simulink model "switch_detect"  (R2023a)
settings: configuration reference "config" (kept outside this file)
model workspace (MAT data in the model file):
  switch_pos = Simulink.Parameter
  switch_pos.Value = 10000
  switch_pos.Description = '开关触发时刻编码器位置'
  switch_pos.DataType = 'int32'
  switch_pos.Complexity = 'real'
  switch_pos.Dimensions = [1 1]
  switch_width = Simulink.Parameter
  switch_width.Value = 10
  switch_width.Description = '开关触发宽度
    | '
  switch_width.DataType = 'int32'
  switch_width.Min = 0
  switch_width.Complexity = 'real'
  switch_width.Dimensions = [1 1]
libraries: servo_hub_lib x1
settings Model: DataDictionary=model_config.sldd  ParameterArgumentNames=switch_pos,switch_width  Creator=huangcheng  LastModifiedBy=Administrator
settings ConfigSetRef: SourceName=config

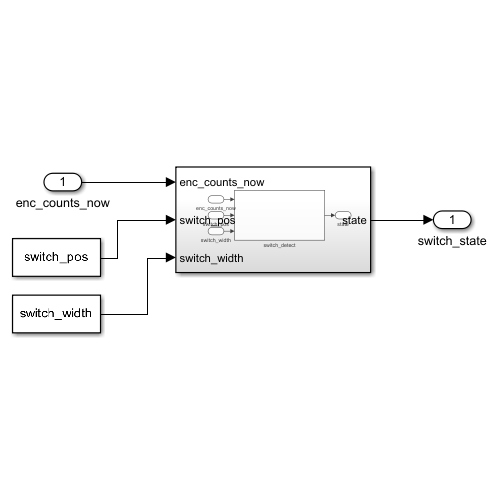
[thumbnail: Simulink's stored preview of the top-level diagram]
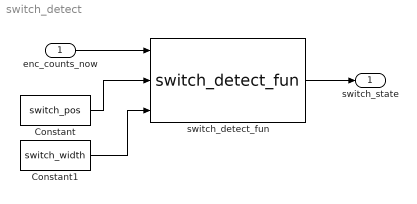
== system switch_detect ==
  enc_counts_now : Inport  OutDataTypeStr=int64
  Constant : Constant  Value=switch_pos  SampleTime=-1
  Constant1 : Constant  Value=switch_width  SampleTime=-1
  switch_detect_fun : servo_hub_lib/fast_math/switch_detect_fun  SystemSampleTime=-1  VariantActivationTime=update diagram  Latency=0  AutoFrameSizeCalculation=off
      settings: SourceProductName=ServoHub Library
  switch_state : Outport
  wires:
  enc_counts_now/1 -> switch_detect_fun/1
  Constant/1 -> switch_detect_fun/2
  Constant1/1 -> switch_detect_fun/3
  switch_detect_fun/1 -> switch_state/1
